simulink model "flightControlSystem"  (R2023b)
settings: Solver=ode3  StartTime=0  StopTime=TFinal  FixedStep=Ts  RelTol=1e-3  EnableMultiTasking=on
undefined symbols (not defined in the file): codertarget, Controller, DiscIntNeverNeededParam, Discrete, Estimator, g, gray, init, orient_ref, pos_ref, Sensors, Time, Ts, var_acc_angle_N, var_bias_gyr_N, var_gyro_p_N, Vehicle
libraries: simulink x46, slpidlib x4, ctrlSharedLib x4, sharedtransform x3, visiontextngfix x3, simulink_extras x1, visionanalysis x1, visiontransforms x1, dspstat3 x1, parrotlib x1
(part 3 of 3)

== matlab function flightControlSystem/Image Processing System/convert to hsv, increase saturation, create colorthresholder mask, ==
  data: R input; I output; G input; B input

function I = fcn(R,G,B)
%createMask  Threshold RGB image using auto-generated code from colorThresholder app.
%  [BW,MASKEDRGBIMAGE] = createMask(RGB) thresholds image RGB using
%  auto-generated code from the colorThresholder app. The colorspace and
%  range for each channel of the colorspace were set within the app. The
%  segmentation mask is returned in BW, and a composite of the mask and
%  original RGB images is returned in maskedRGBImage.

% Auto-generated by colorThresholder app on 10-Jun-2024
%------------------------------------------------------


% Convert RGB image to chosen color space

% Define thresholds for channel 1 based on histogram settings
channel1Min = 203.000;
channel1Max = 255.000;

% Define thresholds for channel 2 based on histogram settings
channel2Min = 202.000;
channel2Max = 255.000;

% Define thresholds for channel 3 based on histogram settings
channel3Min = 203.000;
channel3Max = 255.000;

% Create mask based on chosen histogram thresholds
sliderBW = (R >= channel1Min ) & (R <= channel1Max) & ...
    (G >= channel2Min ) & (G <= channel2Max) & ...
    (B >= channel3Min ) & (B <= channel3Max);
BW = sliderBW;

I = BW;
end

== matlab function flightControlSystem/Control System/Controller/Position Controller/Position error transformation (Earth to Body frame) ==
  data: yaw input; xy_err_earth input; xy_err_body output
function xy_err_body = fcn(yaw,xy_err_earth)

transformation = [cos(yaw), sin(yaw); -sin(yaw),  cos(yaw)];
xy_err_body = transformation * xy_err_earth;


end

== stateflow chart flightControlSystem/Control System/Path Planning/Chart ==
  state NaiveTurning
    entry:
    if lineatleft==1
    turndir=-1;
    elseif lineatright==1
    turndir=1;
    elseif bottomleftturn==0
    turndir=0;
    else turndir=1;
    end
    if linedetected==1
    yawout=yaw+0.005*turndir
    else
    yawout=yaw+0.01*turndir
    end
    during:
    if linedetected==1
    yawout=yaw+0.005*turndir
    else
    yawout=yaw+0.01*turndir
    end
    exit:
    yawout=yaw;
  state PrepareLanding
    entry:
    xtemp=0;
    ytemp=0.5;
    landingy = y+ytemp;
    xout = x + ytemp* sin(yaw) + xtemp*cos(yaw);
    yout = y + ytemp*cos(yaw) - xtemp*sin(yaw);
  state Forward
    entry:
    ytemp = single(0.05 + (circlehigh*0.1)+  (accelerate*0.1) - ((1-ontrack)*(0.05)));
    xout = x + ytemp* sin(yaw) + xtemp*cos(yaw);
    yout = y + ytemp*cos(yaw) - xtemp*sin(yaw);
    end
    during:
    if ~circlehigh
    yawout = yaw + (0.01+ 0.01 * forwardturninglarge)*forwardturning;
    end
    xtemp = (0.005+ 0.02 * forwardturninglarge)*forwardturning;
    ytemp = single(0.05 + (circlehigh*0.05)+  (accelerate*0.1) - ((1-ontrack)*(0.05)));
    % able to turn while moving if angle small enough
    xout = single(x + ytemp* sin(yaw) + xtemp*cos(yaw));
    yout = single(y + ytemp*cos(yaw) - xtemp*sin(yaw));
  state Liftoff
    entry:
    zout=-0.8;
    xtemp=0;
    ytemp=0;
    debug1=0;
    actualturnangle=turnangle;
    during:
    if ~accelerate
    yawout = yaw+0.015;
    end
  state Landing
    entry:
    zout=0;
  (junction 66) -> Forward [order 2] : [ontrack==1]
  Forward -> PrepareLanding [order 1] : [lineatright==0 && lineatright==0 && abs(turnangle)>1.5 && abs(turnangle)<1.65 && circledetector ]
  PrepareLanding -> Landing : [(x-xout)^2+(y-yout)^2<0.02]
  (default) -> Liftoff
  Forward -> NaiveTurning [order 2] : [ontrack == 0]
  Liftoff -> (junction 66) : [z<-0.7]
  (junction 66) -> NaiveTurning [order 1] : [ontrack == 0]
  NaiveTurning -> Forward : [ontrack == 1]
  data: circledetector input; circlehigh input; bottomleftturn input; forwardturninglarge input; ontrack input; z input; x input; y input; turnangle input; yaw input; xout output single; yout output single; zout output; yawout output; accelerate input; linedetected input; forwardturning input; actualturnangle local; lineatright input; lineatleft input; debug1 local; xtemp local single; ytemp local single; turndir local; startingyaw local; remainingangle local; landingy local
